simulink model "PlantTest"  (R2013b)
settings: Solver=ode45  StartTime=0.0  StopTime=5  RelTol=1e-3
values from neighbouring files (symbols this model uses):
  C = C0    [Minimizer.m]    (also in parameters2.m = [1 0 0 0 0 0;0 0 1 0 0 0;0 0 0 0 1 0]; parameters3.m = [1 0 0 0 0 0;0 0 1 0 0 0;0 0 0 0 1 0])
  I = 1/12*M*((2*rx1)^2 + (2*ry1)^2)    (= 7.46230507536)    [BoatController.m]    (also in boatDynamics.m; parameters2.m = 20; parameters3.m)
  M = 80*lbtokg    (= 36.28736)    [BoatController.m]    (also in parameters2.m = 10; parameters3.m)
  rx1 = -12*intom    (= -0.3048)    [BoatController.m]    (also in boatDynamics.m; costfunction.m; parameters3.m)
  rx2 = 12*intom    (= 0.3048)    [BoatController.m]    (also in boatDynamics.m; costfunction.m; parameters3.m)
  ry1 = -69*intom/2 + 6*intom    (= -0.7239)    [BoatController.m]    (also in boatDynamics.m; costfunction.m; parameters3.m)
  ry2 = ry1    (= -0.7239)    [BoatController.m]    (also in boatDynamics.m; costfunction.m; parameters3.m)
settings Model: Creator=darsan13  LastModifiedBy=darsan13

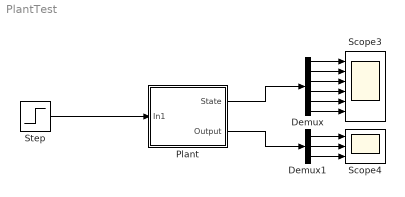
== system PlantTest ==
  Demux : Demux  Outputs=6
  Demux1 : Demux  Outputs=3
  Plant : Subsystem  mask{rx1=rx1, rx2=rx2, ry1=ry1, ry2=ry2, M=M, I=I, C=C}
      mask TypeOptions rx1: Constant/Value
  Scope3 : Scope  NumInputPorts=6
      settings: YMin=-250000~-4.5~-5~-5~-5~-5  YMax=250000~4.5~5~5~5~5
  Scope4 : Scope  NumInputPorts=3
      settings: YMin=-250000~-4.5~-5  YMax=250000~4.5~5
  Step : Step  Before=[0;0;0;0]  After=|  SampleTime=0
      | [0;
      | 10; 0; 10]
  wires:
  Demux/1 -> Scope3/1
  Demux/2 -> Scope3/2
  Demux/3 -> Scope3/3
  Demux/4 -> Scope3/4
  Demux/5 -> Scope3/5
  Demux/6 -> Scope3/6
  Plant/1(State) -> Demux/1
  Plant/2(Output) -> Demux1/1
  Demux1/1 -> Scope4/1
  Demux1/2 -> Scope4/2
  Demux1/3 -> Scope4/3
  Step/1 -> Plant/1(In1)

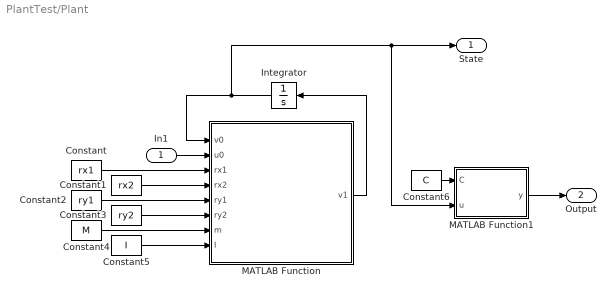
== system PlantTest/Plant ==
  In1 : Inport
  Constant : Constant  Value=rx1
  Constant1 : Constant  Value=rx2
  Constant2 : Constant  Value=ry1
  Constant3 : Constant  Value=ry2
  Constant4 : Constant  Value=M
  Constant5 : Constant  Value=I
  Constant6 : Constant  Value=C
  Integrator : Integrator  InitialCondition=[0 0 0 0 90 0]
  MATLAB Function : MATLAB Function  TreatAsAtomicUnit=on
  MATLAB Function1 : MATLAB Function  TreatAsAtomicUnit=on
  State : Outport
  Output : Outport  Port=2
  wires:
  MATLAB Function1/1(y) -> Output/1
  Constant6/1 -> MATLAB Function1/1(C)
  In1/1 -> MATLAB Function/2(u0)
  Integrator/1 -> MATLAB Function1/2(u), State/1, MATLAB Function/1(v0)
  MATLAB Function/1(v1) -> Integrator/1
  Constant5/1 -> MATLAB Function/8(I)
  Constant4/1 -> MATLAB Function/7(m)
  Constant3/1 -> MATLAB Function/6(ry2)
  Constant2/1 -> MATLAB Function/5(ry1)
  Constant1/1 -> MATLAB Function/4(rx2)
  Constant/1 -> MATLAB Function/3(rx1)

== matlab function PlantTest/Plant/MATLAB Function ==
  data: v0 input; v1 output; u0 input; rx1 input; rx2 input; ry1 input; ry2 input; m input; I input
function v1   = boatDynamics(v0, u0, rx1, rx2, ry1, ry2, m, I)

    % %%%%%%%%%%%%%%%%%%%%%%%%%%%%%%%%%%%%%%%%%%%% %
    %    v = [x...          %    u = [theta1...    %
    %        x_dot...       %        f1...         %
    %        y...           %        theta2...     %
    %        y_dot...       %        f2]           %
    %        theta...       %                      %
    %        theta_dot];    %                      %
    % %%%%%%%%%%%%%%%%%%%%%%%%%%%%%%%%%%%%%%%%%%%% %
    
    v11 = v0(2);
    v12 = -u0(2)/m*sind(u0(1)+v0(5)) - u0(4)/m*sind(u0(3)+v0(5)) - 0*5*v0(1);
    v13 = v0(4);
    v14 = u0(2)/m*cosd(u0(1)+v0(5)) + u0(4)/m*cosd(u0(3)+v0(5)) - 0*2*v0(3);
    v15 = v0(6);
    v16 = rx1/I*u0(2)*cosd(u0(1)) + ry1/I*u0(2)*sind(u0(1)) + rx2/I*u0(4)*cosd(u0(3)) + ry2/I*u0(4)*sind(u0(3)) - 0*9*v0(5);
   
    v1 = [v11;v12;v13;v14;v15;v16];
    
    
end

== matlab function PlantTest/Plant/MATLAB Function1 ==
  data: C input; u input; y output
function y = fcn(C,u)
%#codegen

y = C*u;
